simulink model "BBB_I2C_Write_Test_LibraryBlock"  (R2013a)
settings: Solver=FixedStepDiscrete  StartTime=0.0  StopTime=inf  RelTol=1e-3
libraries: BLACKlink x2, simulink x2
settings Model: SimulationMode=external  ExtModeTrigDuration=100  Creator=rdustinkahawita  LastModifiedBy=rdustinkahawita
settings OptimizationCC: OptimizeModelRefInitCode=on  LifeSpan=1
settings DebuggingCC: SolverPrmCheckMsg=none  StrictBusMsg=Warning
settings HardwareCC: ProdLargestAtomicInteger=Long  ProdLargestAtomicFloat=Double  ProdEndianess=LittleEndian  ProdHWDeviceType=ARM Compatible->ARM Cortex
settings RTWCC: SystemTargetFile=realtime.tlc  GenerateMakefile=off  TemplateMakefile=realtime.tmf  Description=Run on Target Hardware  RTWVerbose=off  ProcessScript=realtime_make_rtw_hook
settings STFCustomTargetCC: TargetLibSuffix=.a  GenerateSampleERTMain=on  ERTCustomFileBanners=on  SupportNonInlinedSFcns=off  SupportVariableSizeSignals=on  MATLABClassNameForMDSCustomization=Simulink.SoftwareTarget.ERTCustomization  SystemTargetFile=realtime.tlc
settings ERTTargetCC: ParMdlRefBuildCompliant=off  CompOptLevelCompliant=off  ConcurrentExecutionCompliant=off  CombineOutputUpdateFcns=off  ERTFirstTimeCompliant=off  SupportContinuousTime=on  SupportVariableSizeSignals=on  ModelStepFunctionPrototypeControlCompliant=off  CPPClassGenCompliant=off  ExtMode=on  ExtModeMexArgs='192.168.7.2' 0 17725  ERTSrcFileBannerTemplate=realtime_code_template.cgt  ERTHdrFileBannerTemplate=realtime_code_template.cgt  ERTDataSrcFileTemplate=realtime_code_template.cgt  ERTDataHdrFileTemplate=realtime_code_template.cgt  ERTCustomFileTemplate=realtime_file_process.tlc

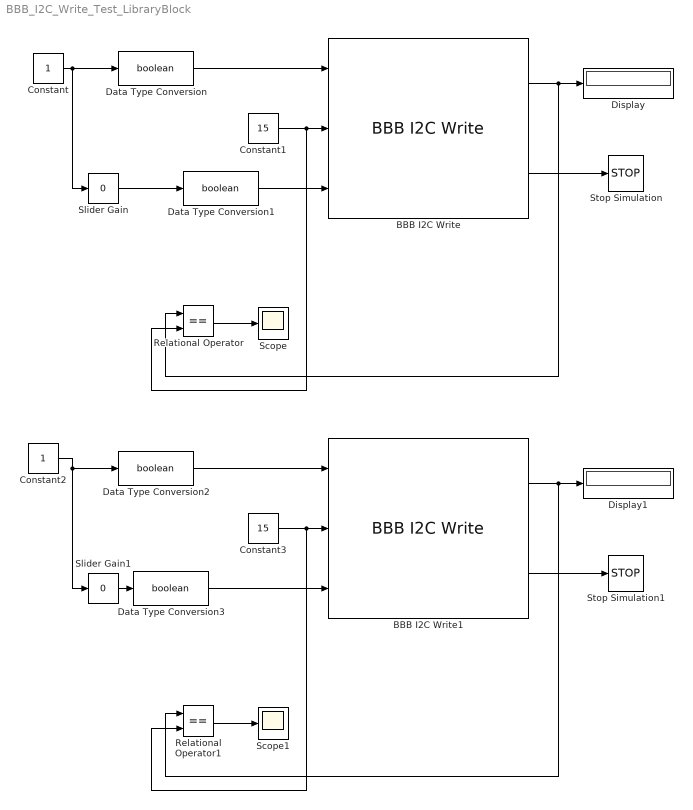
== system BBB_I2C_Write_Test_LibraryBlock ==
  BBB I2C Write : BLACKlink/BBB I2C Write  BBB_I2CBusNo=BeagleBone Black I2C Channel 1  BBB_I2CAddress=104  BBB_I2CRegister=32  BBB_DebugInfo=Debug Level 4 - Include Device Registery Read-Out
  BBB I2C Write1 : BLACKlink/BBB I2C Write  BBB_I2CBusNo=BeagleBone Black I2C Channel 1  BBB_I2CAddress=104  BBB_I2CRegister=32  BBB_DebugInfo=Debug Level 4 - Include Device Registery Read-Out
  Constant : Constant
  Constant1 : Constant  Value=15  OutDataTypeStr=uint8
  Constant2 : Constant
  Constant3 : Constant  Value=15  OutDataTypeStr=uint8
  Data Type Conversion{,1..3} (4 alike) : DataTypeConversion  OutMin=[0]  OutMax=[1]  OutDataTypeStr=boolean
  Display : Display
      settings: Format=hex (Stored Integer)
  Display1 : Display
      settings: Format=hex (Stored Integer)
  Relational Operator : RelationalOperator  Operator===  OutDataTypeStr=boolean
  Relational Operator1 : RelationalOperator  Operator===  OutDataTypeStr=boolean
  Scope : Scope
      settings: TimeRange=60
  Scope1 : Scope
  Slider Gain : simulink/Math Operations/Slider Gain  low=0  gain=0  high=1
  Slider Gain1 : simulink/Math Operations/Slider Gain  low=0  gain=0  high=1
  Stop Simulation : Stop
  Stop Simulation1 : Stop
  wires:
  Constant/1 -> Slider Gain/1, Data Type Conversion/1
  Slider Gain/1 -> Data Type Conversion1/1
  Data Type Conversion/1 -> BBB I2C Write/1
  Constant1/1 -> Relational Operator/2, BBB I2C Write/2
  BBB I2C Write/1 -> Relational Operator/1, Display/1
  Relational Operator/1 -> Scope/1
  Data Type Conversion1/1 -> BBB I2C Write/3
  BBB I2C Write/2 -> Stop Simulation/1
  Constant2/1 -> Slider Gain1/1, Data Type Conversion2/1
  Slider Gain1/1 -> Data Type Conversion3/1
  Data Type Conversion2/1 -> BBB I2C Write1/1
  Constant3/1 -> Relational Operator1/2, BBB I2C Write1/2
  BBB I2C Write1/1 -> Relational Operator1/1, Display1/1
  Relational Operator1/1 -> Scope1/1
  Data Type Conversion3/1 -> BBB I2C Write1/3
  BBB I2C Write1/2 -> Stop Simulation1/1
